simulink model "robust_test_sim"  (R2022b)
settings: Solver=FixedStepAuto  StartTime=0.0  StopTime=time_final  RelTol=1e-3  EnableMultiTasking=on
values from neighbouring files (symbols this model uses):
  Stepsize = 0.4    [performance_test.m]    (also in robust_test.m; step_response_our.m = 0)
  time_final = 20    [performance_test.m]    (also in robust_test.m)
  Ts = Ts_all(2)    [performance_test.m]    (also in robust_plot.m = Ts_all(ii); robust_test.m; step_response_our.m = TS(i))
undefined symbols (not defined in the file or in its folder): A_d, B_d, C_d, K_SF, L_Pred, N
settings Model: ExtModeTrigDuration=8  Creator=Alex Zhen  LastModifiedBy=Alex Zhen
settings OptimizationCC: DefaultUnderspecifiedDataType=single  EnhancedBackFolding=on  PassReuseOutputArgsAs=Individual arguments  MaxStackSize=1024  OptimizeBlockOrder=speed  DifferentSizesBufferReuse=on  OptimizationCustomize=off  DenormalBehavior=FlushToZero  EfficientTunableParamExpr=on
settings DebuggingCC: ParameterTunabilityLossMsg=error
settings HardwareCC: ProdBitPerChar=16  ProdBitPerInt=16  ProdBitPerPointer=32  ProdBitPerSizeT=32  ProdBitPerPtrDiffT=32  ProdLargestAtomicInteger=Integer  ProdLargestAtomicFloat=None  ProdWordSize=16  ProdLongLongMode=on  ProdHWDeviceType=Texas Instruments->C2000
settings SFSimCC: MATLABDynamicMemAlloc=off
settings RTWCC: Description=Embedded Coder  SystemTargetFile=ert.tlc  HardwareBoard=TI Delfino F28379D LaunchPad  TLCOptions=-aInlineSetEventsForThisBaseRateFcn=TLC_FALSE -aSuppressMultiTaskScheduler=TLC_FALSE -aRateBasedStepFcn=1  TemplateMakefile=ert_default_tmf  Toolchain=Texas Instruments Code Composer Studio (C2000)
settings CodeAppCC: ForceParamTrailComments=on  IgnoreCustomStorageClasses=off  OperatorAnnotations=on  SimulinkDataObjDesc=on  SFDataObjDesc=on  InsertBlockDesc=on
settings ERTTargetCC: CodeReplacementLibrary=TI C28x  SupportContinuousTime=on  ExtModeTransport=4  ExtModeStaticAlloc=on  ExtModeAutomaticAllocSize=off  ExtModeMexFile=ext_xcp  ExtModeIntrfLevel=Level2 - Open

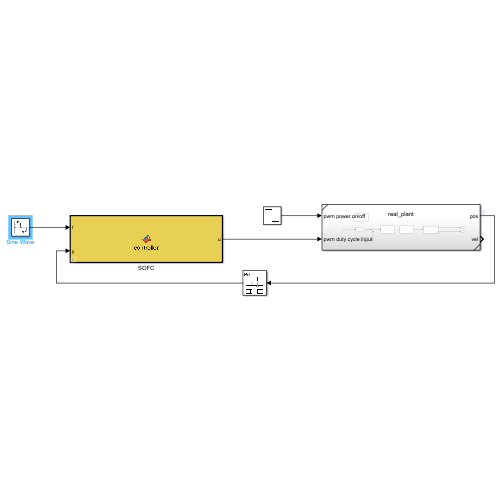
[thumbnail: Simulink's stored preview of the top-level diagram]
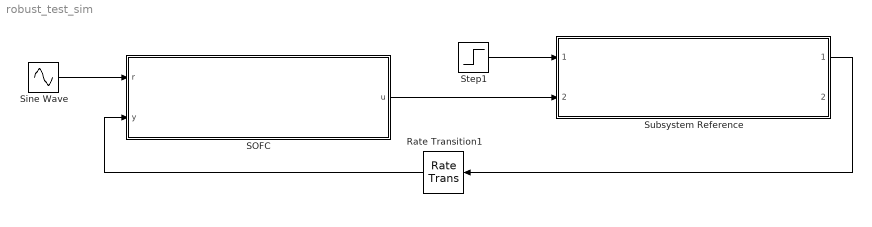
== system robust_test_sim ==
  Rate Transition1 : RateTransition  Deterministic=off  OutPortSampleTime=Ts
  SOFC : MATLAB Function  TreatAsAtomicUnit=on  mask{A=A_d, B=B_d, C=C_d, K=K_SF, L=L_Pred, N=N}
  Sine Wave : Sin  Amplitude=Stepsize  Bias=Stepsize/2  Frequency=3*pi  SampleTime=Ts
  Step1 : Step  Time=time_final  Before=1  After=0  SampleTime=0
  Subsystem Reference : Subsystem  ReferencedSubsystem=real_plant
  wires:
  Subsystem Reference/1 -> Rate Transition1/1
  Step1/1 -> Subsystem Reference/1
  SOFC/1(u) -> Subsystem Reference/2
  Rate Transition1/1 -> SOFC/2(y)
  Sine Wave/1 -> SOFC/1(r)

== matlab function robust_test_sim/SOFC ==
  data: r input; u output; y input; A parameter; B parameter; C parameter; K parameter; L parameter; N parameter
function u = controller(r, y,A, B, C, K, L, N)
n = size(A,1);
persistent xhat;  %memory for the state
  if isempty(xhat)  %local variable initialization
        xhat=zeros(n,1);   
  end

u = -K*xhat+N*r; %Control computation
u_unsat = -K*xhat+N*r; %Control computation with integral action 
u= sign(u_unsat)*min(1,abs(u_unsat));
%DAC(u) send out control here to minimize computation delay
%Update the next state next
xhat = (A-L*C)*xhat + B*u + L*y;
